simulink model "DegradationParameterBuckConverter"  (R2021a)
settings: Solver=VariableStepAuto  StartTime=0.0  StopTime=10.0  RelTol=1e-3
values from neighbouring files (symbols this model uses):
  buck_Fsw_M_adjustment = -0.2    [Run_GeneratorRectifierBuckConverterModel.m]
  buck_TFall_M_adjustment = -0.2    [Run_GeneratorRectifierBuckConverterModel.m]
  buck_Trr_M_adjustment = -0.2    [Run_GeneratorRectifierBuckConverterModel.m]
undefined symbols (not defined in the file or in its folder): buck_TRise_M_adjustment
libraries: Lib_EMTAT x5
settings Model: Creator=sfaulk  LastModifiedBy=mebell

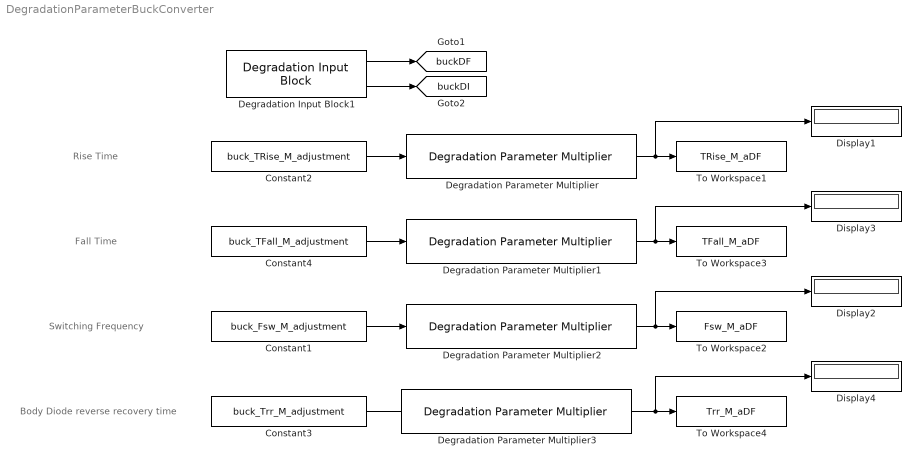
== system DegradationParameterBuckConverter ==
  note: Rise Time
  note: Fall Time
  note: Switching Frequency
  note: Body Diode reverse recovery time
  Constant1 : Constant  Value=buck_Fsw_M_adjustment
  Constant2 : Constant  Value=buck_TRise_M_adjustment
  Constant3 : Constant  Value=buck_Trr_M_adjustment
  Constant4 : Constant  Value=buck_TFall_M_adjustment
  Degradation Input Block1 : Lib_EMTAT/Components/Physics-Based/Degradation Input Block  SystemSampleTime=-1  VariantActivationTime=update diagram  Latency=0  AutoFrameSizeCalculation=off
      settings: SourceProductName=EMTAT
  Degradation Parameter Multiplier{,1..3} (4 alike) : Lib_EMTAT/Components/Physics-Based/Degradation Parameter Multiplier  SystemSampleTime=-1  VariantActivationTime=update diagram  Latency=0  AutoFrameSizeCalculation=off
      settings: SourceProductName=EMTAT
  Display{1..4} (4 alike) : Display
  To Workspace1 : ToWorkspace  VariableName=TRise_M_aDF  SaveFormat=Timeseries  SampleTime=-1
      settings: Save2DSignal=2-D array (concatenate along first dimension)
  To Workspace2 : ToWorkspace  VariableName=Fsw_M_aDF  SaveFormat=Timeseries  SampleTime=-1
      settings: Save2DSignal=2-D array (concatenate along first dimension)
  To Workspace3 : ToWorkspace  VariableName=TFall_M_aDF  SaveFormat=Timeseries  SampleTime=-1
      settings: Save2DSignal=2-D array (concatenate along first dimension)
  To Workspace4 : ToWorkspace  VariableName=Trr_M_aDF  SaveFormat=Timeseries  SampleTime=-1
      settings: Save2DSignal=2-D array (concatenate along first dimension)
  tag scope: buckDF=global, buckDI=global
  wires:
  Degradation Input Block1/2 -> [buckDI]
  Degradation Input Block1/1 -> [buckDF]
  Degradation Parameter Multiplier/1 -> Display1/1, To Workspace1/1
  Constant2/1 -> Degradation Parameter Multiplier/1
  Constant4/1 -> Degradation Parameter Multiplier1/1
  Degradation Parameter Multiplier1/1 -> Display3/1, To Workspace3/1
  Constant1/1 -> Degradation Parameter Multiplier2/1
  Degradation Parameter Multiplier2/1 -> Display2/1, To Workspace2/1
  Constant3/1 -> ?
  Degradation Parameter Multiplier3/1 -> Display4/1, To Workspace4/1
